simulink model "Levitatore_mdl"  (Simulink 7.2)
settings: Solver=ode45  StartTime=0.0  StopTime=10.0  RelTol=1e-3
values from neighbouring files (symbols this model uses):
  dx0 = 0    [TSC160127ProvaMatlab.m]
  g = 9.81    [TSC160127ProvaMatlab.m]
  k0 = 4    [TSC160127ProvaMatlab.m]
  km = 5    [TSC160127ProvaMatlab.m]
  kv = 1    [TSC160127ProvaMatlab.m]
  m = 5    [TSC160127ProvaMatlab.m]
  v0 = 2    [TSC160127ProvaMatlab.m]
  x0 = 0.5 + 0.03    (= 0.53)    [TSC160127ProvaMatlab.m]
undefined symbols (not defined in the file or in its folder): magnitude
settings Model: Creator=lbiagiotti  LastModifiedBy=lbiagiotti
settings OptimizationCC: InlineParams=on

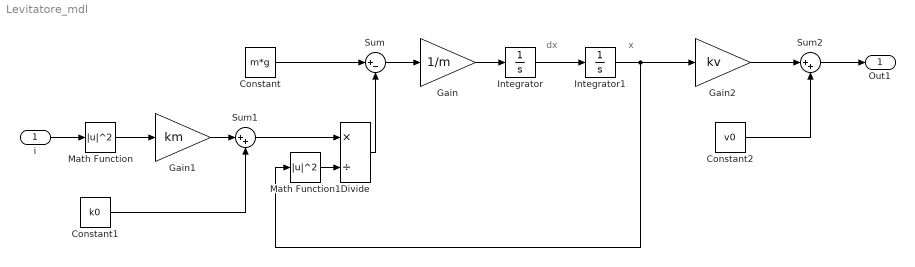
== system Levitatore_mdl ==
  note: dx
  note: x
  i : Inport  OutDataType=sfix(16)  OutScaling=2^0
  Constant : Constant  Value=m*g  OutDataType=sfix(16)  OutScaling=2^0
  Constant1 : Constant  Value=k0  OutDataType=sfix(16)  OutScaling=2^0
  Constant2 : Constant  Value=v0  OutDataType=sfix(16)  OutScaling=2^0
  Divide : Product  Inputs=*/  OutDataType=sfix(16)  OutScaling=2^-10
  Gain : Gain  Gain=1/m  ParameterDataType=sfix(16)  ParameterScaling=2^0  OutDataType=sfix(16)  OutScaling=2^0
  Gain1 : Gain  Gain=km  ParameterDataType=sfix(16)  ParameterScaling=2^0  OutDataType=sfix(16)  OutScaling=2^0
  Gain2 : Gain  Gain=kv  ParameterDataType=sfix(16)  ParameterScaling=2^0  OutDataType=sfix(16)  OutScaling=2^0
  Integrator : Integrator  InitialCondition=dx0
  Integrator1 : Integrator  InitialCondition=x0
  Math Function : Math  Operator=magnitude^2  OutDataType=sfix(16)  OutScaling=2^0  SaturateOnIntegerOverflow=on
  Math Function1 : Math  Operator=magnitude^2  OutDataType=sfix(16)  OutScaling=2^0  SaturateOnIntegerOverflow=on
  Sum : Sum  Inputs=|+-  OutDataType=sfix(16)  OutScaling=2^0
  Sum1 : Sum  Inputs=|++  OutDataType=sfix(16)  OutScaling=2^0
  Sum2 : Sum  Inputs=|++  OutDataType=sfix(16)  OutScaling=2^0
  Out1 : Outport  OutDataType=sfix(16)  OutScaling=2^0
  wires:
  Constant/1 -> Sum/1
  Math Function/1 -> Gain1/1
  Gain1/1 -> Sum1/1
  Constant1/1 -> Sum1/2
  Sum1/1 -> Divide/1
  Integrator/1 -> Integrator1/1
  Divide/1 -> Sum/2
  Integrator1/1 -> Gain2/1, Math Function1/1
  Sum/1 -> Gain/1
  Gain/1 -> Integrator/1
  Gain2/1 -> Sum2/1
  Constant2/1 -> Sum2/2
  Sum2/1 -> Out1/1
  Math Function1/1 -> Divide/2
  i/1 -> Math Function/1
